simulink model "softarm_actuator_force_block"  (R2025a)
settings: Solver=ode15s  StartTime=0.0  StopTime=1  RelTol=1e-3
PreLoadFcn:
  | softarm_root=fileparts(get_param(bdroot,'FileName'));addpath(softarm_root);addpath(fullfile(softarm_root,'matlab'));
InitFcn:
  | softarm_root=fileparts(get_param(bdroot,'FileName'));addpath(fullfile(softarm_root,'matlab'));if evalin('base','exist(''softarm_bundle'',''var'')'),softarm_selected_bundle=evalin('base','softarm_bundle');else,softarm_selected_bundle=fullfile(softarm_root,'examples','generated','pcc_three_tendon_extensible_n2');end;softarm_loaded=softarm.initModel(string(softarm_selected_bundle));assert(~isempty(softarm_loaded.actuation),'softarm:MissingActuation','Selected bundle has no actuator mapping.');
undefined symbols (not defined in the file or in its folder): softarm_p
settings Model: Creator=rlwan  LastModifiedBy=rlwan

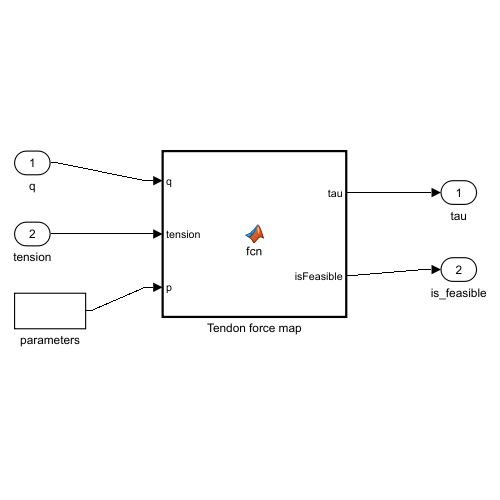
[thumbnail: Simulink's stored preview of the top-level diagram]
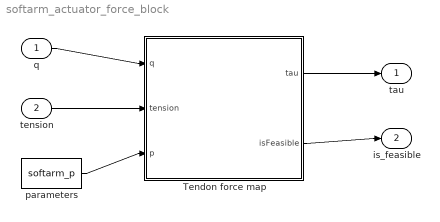
== system softarm_actuator_force_block ==
  q : Inport  PortDimensions=softarm_nq
  tension : Inport  Port=2  PortDimensions=softarm_nu
  Tendon force map : MATLAB Function  TreatAsAtomicUnit=on
  parameters : Constant  Value=softarm_p
  tau : Outport
  is_feasible : Outport  Port=2
  wires:
  q/1 -> Tendon force map/1(q)
  tension/1 -> Tendon force map/2(tension)
  parameters/1 -> Tendon force map/3(p)
  Tendon force map/1(tau) -> tau/1
  Tendon force map/2(isFeasible) -> is_feasible/1

== matlab function softarm_actuator_force_block/Tendon force map ==
  data: q input; tau output; tension input; p input; isFeasible output
function [tau,isFeasible] = fcn(q,tension,p)
%#codegen
[tau,isFeasible]=softarm_actuator_force(q,tension,p);
end
